simulink model "LIFT"  (R2019b)
settings: Solver=VariableStepAuto  StartTime=0.0  StopTime=inf  RelTol=1e-3
settings Model: Creator=u1830311  LastModifiedBy=u1830311

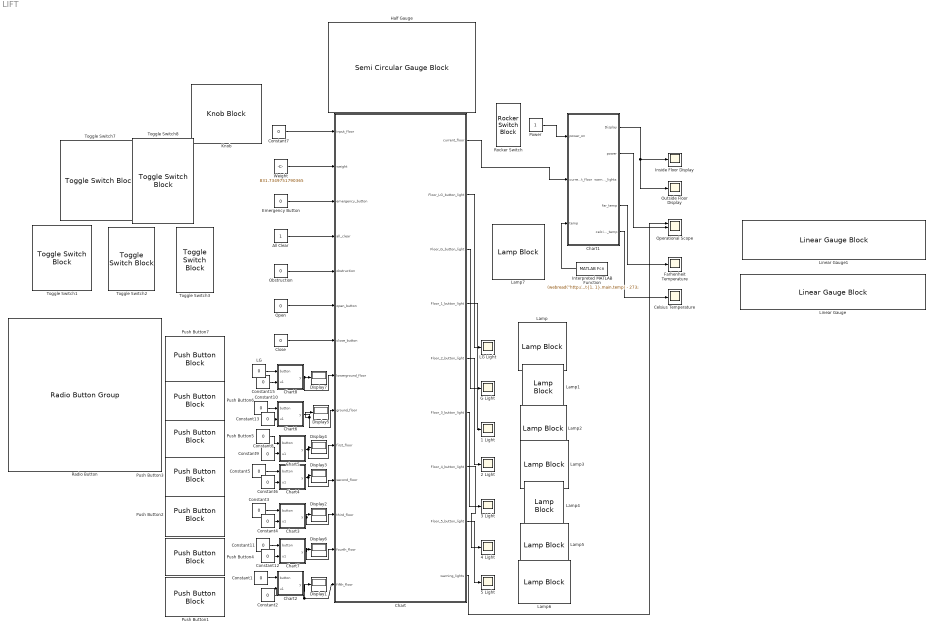
== system LIFT ==
  1 Light : Scope
  2 Light : Scope
  3 Light : Scope
  4 Light : Scope
  5 Light : Scope
  All Clear : Constant
  Celsius Temperature : Scope
  Chart : Stateflow chart  TreatAsAtomicUnit=on
  Chart1 : Stateflow chart  BlockKeywords=__PRM__SERIALIZED__DATA__:Stateflow Chart,Stateflow Diagram  TreatAsAtomicUnit=on
  Chart2 : Stateflow chart  BlockKeywords=__PRM__SERIALIZED__DATA__:Stateflow Chart,Stateflow Diagram  TreatAsAtomicUnit=on
  Chart3 : Stateflow chart  BlockKeywords=__PRM__SERIALIZED__DATA__:Stateflow Chart,Stateflow Diagram  TreatAsAtomicUnit=on
  Chart4 : Stateflow chart  BlockKeywords=__PRM__SERIALIZED__DATA__:Stateflow Chart,Stateflow Diagram  TreatAsAtomicUnit=on
  Chart5 : Stateflow chart  BlockKeywords=__PRM__SERIALIZED__DATA__:Stateflow Chart,Stateflow Diagram  TreatAsAtomicUnit=on
  Chart6 : Stateflow chart  BlockKeywords=__PRM__SERIALIZED__DATA__:Stateflow Chart,Stateflow Diagram  TreatAsAtomicUnit=on
  Chart7 : Stateflow chart  BlockKeywords=__PRM__SERIALIZED__DATA__:Stateflow Chart,Stateflow Diagram  TreatAsAtomicUnit=on
  Chart8 : Stateflow chart  BlockKeywords=__PRM__SERIALIZED__DATA__:Stateflow Chart,Stateflow Diagram  TreatAsAtomicUnit=on
  Close : Constant  Value=0
  Constant{1..13,15} (14 alike) : Constant  Value=0
  Display{1..7} (7 alike) : Display
  Emergency Button : Constant  Value=0
  Farhenheit Temperature : Scope
  G Light : Scope
  Half Gauge : SemiCircularGaugeBlock  ScaleMin=-1  ScaleMax=5  TickInterval=1
  "Inside Floor Display " : Scope
  Interpreted MATLAB Function : MATLABFcn  MATLABFcn="(webread(\"http://api.openweathermap.org/data/2.5/forecast?id=2652221&APPID=0d4add3479401fba2717516fc46e760f\").list{1, 1}.main.temp) - 273;"  OutputDimensions=1
  Knob : KnobBlock  ScaleMax=2000
  LG : Constant  Value=0
  LG Light : Scope
  Lamp{,1..7} (8 alike) : LampBlock
  Linear Gauge : LinearGaugeBlock  ScaleMin=-10  ScaleMax=50
  Linear Gauge1 : LinearGaugeBlock  ScaleMin=14  ScaleMax=122
  Obstruction : Constant  Value=0
  Open : Constant  Value=0
  "Operational Scope " : Scope  NumInputPorts=3
  "Outside Floor Display " : Scope
  Power : Constant
  Push Button1 : PushButtonBlock  ButtonText=5
  Push Button2 : PushButtonBlock  ButtonText=3
  Push Button3 : PushButtonBlock  ButtonText=2
  Push Button4 : PushButtonBlock  ButtonText=4
  Push Button5 : PushButtonBlock  ButtonText=1
  Push Button6 : PushButtonBlock  ButtonText=G
  Push Button7 : PushButtonBlock  ButtonText=LG
  Radio Button : RadioButtonGroup  SelectedLabel=Ground  ButtonGroupName=Start Floor
      settings: Values={{'Lower Ground', 'Ground', '1', '2', '3', '4', '5'}, [-1 0 1 2 3 4 5]}
  Rocker Switch : RockerSwitchBlock
      settings: Values={{'Off', 'On'}, [0 1]}
  Toggle Switch{1..3,7..8} (5 alike) : ToggleSwitchBlock
      settings: Values={{'Off', 'On'}, [0 1]}
  "Weight " : Constant  Value=831.7349751790365
  wires:
  Chart/1(current_floor) -> Chart1/2(current_floor)
  Constant7/1 -> Chart/1(input_floor)
  Power/1 -> Chart1/1(power_on)
  Chart1/2(power) -> "Operational Scope "/2
  Chart1/1(Display) -> "Outside Floor Display "/1, "Inside Floor Display "/1
  Chart1/4(far_temp) -> Farhenheit Temperature/1
  Chart1/5(celcius_temp) -> Celsius Temperature/1
  Chart/4(Floor_1_button_light) -> 1 Light/1
  Chart/5(Floor_2_button_light) -> 2 Light/1
  Chart/6(Floor_3_button_light) -> 3 Light/1
  Chart/7(Floor_4_button_light) -> 4 Light/1
  Chart/8(Floor_5_button_light) -> 5 Light/1
  All Clear/1 -> Chart/4(all_clear)
  "Weight "/1 -> Chart/2(weight)
  Emergency Button/1 -> Chart/3(emergency_button)
  Chart/9(warning_lights) -> "Operational Scope "/1
  Chart/3(Floor_G_button_light) -> G Light/1
  Chart/2(Floor_LG_button_light) -> LG Light/1
  Constant11/1 -> Chart7/1(button)
  Chart7/1(y) -> Display6/1, Chart/13(fourth_floor)
  Constant12/1 -> Chart7/2(u1)
  Constant2/1 -> Chart2/2(u1)
  Chart2/1(y) -> Display1/1, Chart/14(fifth_floor)
  Constant1/1 -> Chart2/1(button)
  Chart3/1(y) -> Display2/1, Chart/12(third_floor)
  Constant4/1 -> Chart3/2(u1)
  Constant3/1 -> Chart3/1(button)
  Chart4/1(y) -> Display3/1, Chart/11(second_floor)
  Constant6/1 -> Chart4/2(u1)
  Constant5/1 -> Chart4/1(button)
  Chart5/1(y) -> Chart/10(first_floor), Display4/1
  Constant8/1 -> Chart5/1(button)
  Chart6/1(y) -> Display5/1, Chart/9(ground_floor)
  Constant13/1 -> Chart6/2(u1)
  Constant10/1 -> Chart6/1(button)
  Chart8/1(y) -> Chart/8(lowerground_floor), Display7/1
  Constant15/1 -> Chart8/2(u1)
  LG/1 -> Chart8/1(button)
  Constant9/1 -> Chart5/2(u1)
  Obstruction/1 -> Chart/5(obstruction)
  Close/1 -> Chart/7(close_button)
  Open/1 -> Chart/6(open_button)
  Interpreted MATLAB Function/1 -> Chart1/3(temp)

== stateflow chart LIFT/Chart ==
  state Update_F2
    Floors(4) = 1;
  state Update_F4
    Floors(6) = 1;
  state Update_G
    Floors(2) = 1;
  state Update_F1
    Floors(3) = 1;
  state Update_F3
    Floors(5) = 1;
  state Update_F5
    Floors(7) = 1;
  state Update_LG
    Floors(1) = 1;
  state Moving
    entry:
    music=1;
    disp("music plays")
    during:
    if emergency_button == 1 || weight >= 1500
    emergency = 1;
    end
    state Up
      entry:
      if Floors(1)==1
      Floor_LG_button_light=1;
      end
      if Floors(2)==1
      Floor_G_button_light=1;
      end
      if Floors(3)==1
      Floor_1_button_light=1;
      end
      if Floors(4)==1
      Floor_2_button_light=1;
      end
      if Floors(5)==1
      Floor_3_button_light=1;
      end
      if Floors(6)==1
      Floor_4_button_light=1;
      end
      if Floors(7)==1
      Floor_5_button_light=1;
      end
      move=0;
      i=1;
      for(j=(current_floor+2):1:7)
      if (Floors(j)==1)
      up=1;
      break
      else
      up=0;
      end
      end
      during:
      for(j=(current_floor+2):1:7)
      if (Floors(j)==1)
      up=1;
      break
      else
      up=0;
      end
      end
      for (l=-1:1:4)
      while current_floor==l
      for(i=current_floor+2:1:7)
      if(Floors(i)==1)
      move=1;
      break
      end
      end
      break
      end
      end
    state Down
      entry:
      move=0;k=7;
      for(j=(current_floor+2):1:1)
      if (Floors(j)==1)
      up=0;
      break
      else
      up=1;
      end
      end
      during:
      for(m=5:-1:0)
      while current_floor==m
      for(k=current_floor+2:-1:1)
      if(Floors(k)==1)
      move=1;
      break
      end
      end
      break
      end
      end
    state Transport
      entry:
      if up==1
      current_floor=i-2;
      else
      current_floor=k-2;
      end
      if current_floor==-1
      Floor_LG_button_light=0;
      elseif current_floor==0
      Floor_G_button_light=0;
      elseif current_floor==1
      Floor_1_button_light=0;
      elseif current_floor==2
      Floor_2_button_light=0;
      elseif current_floor==3
      Floor_3_button_light=0;
      elseif current_floor==4
      Floor_4_button_light=0;
      elseif current_floor==5
      Floor_5_button_light=0;
      end
      exit:
      if up==1
      Floors(i)=0;
      else
      Floors(k)=0;
      end
      state Open_door
        entry:
        door_state=1;
        music = 0;
        sound = 1;
        switch current_floor
        case (-1)
        disp("Announcer: lower ground floor")
        disp("opening lower ground doors")
        case 0
        disp("Announcer: ground floor")
        disp("opening ground floor doors")
        case 1
        disp("Announcer: floor 1")
        disp("opening floor 1 doors")
        case 2
        disp("Announcer: floor 2")
        disp("opening floor 2 doors")
        case 3
        disp("Announcer: floor 3")
        disp("opening floor 3 doors")
        case 4
        disp("Announcer: floor 4")
        disp("opening floor 4 doors")
        case 5
        disp("Announcer: floor 5")
        disp("opening floor 5 doors")
        end
        sound = 0;
        pause(1)
        if door_state == 1
        disp("doors opening ")
        end
        during:
        tic
        while (toc<10)
        if obstruction == 1
        break
        end
        if close_button == 1
        break
        end
        if open_button == 1
        break
        end
        end
        exit:
      state Idle1
        entry:
        pause(3);
        door_state = 1;
        move=0;
      state Close_Door
        % Closes door
        during:
        pause(3);
        door_state = 0;
        sound = 1;
        if door_state == 0
        disp("Announcer: doors closing")
        switch current_floor
        case (-1)
        disp("system.out closing lower ground doors")
        case 0
        disp("system.out closing ground floor doors")
        case 1
        disp("system.out closing floor 1 doors")
        case 2
        disp("system.out closing floor 2 doors")
        case 3
        disp("system.out closing floor 3 doors")
        case 4
        disp("system.out closing floor 4 doors")
        case 5
        disp("system.out closing floor 5 doors")
        end
        end
        pause(2)
        music = 1;
        disp("music plays")
      (default) -> Idle1
      Idle1 -> Open_door : [move == 0]
      Open_door -> Open_door [order 1] : [open_button == 1 || obstruction == 1]
      Open_door -> Close_Door [order 2] : [(obstruction == 0 && open_button == 0) || close_button == 1]
    (default) -> Up
    Up -> Down [order 1] : [up==0]
    Down -> Up [order 1] : [up==1]
    Down -> Transport [order 2] : [move==1]
    Transport -> Down [order 2] : [move==0&&up==0&&door_state==0]
    Up -> Transport [order 2] : [move==1]
    Transport -> Up [order 1] : [move==0&&up==1&&door_state==0]
  state Input
    entry:
    Floors=[ lowerground_floor ground_floor first_floor second_floor third_floor fourth_floor fifth_floor ]'
    current_floor=input_floor;
    emergency = 0;
    Original=Floors
    during:
    Floors=[ lowerground_floor ground_floor first_floor second_floor third_floor fourth_floor fifth_floor ]'
  state Idle
    entry:
    music=0;
    door_state=1;
    exit:
    door_state=0;
    during:
    if [Floors(1)==0&&Floors(2)==0&&Floors(3)==0&&Floors(4)==0&&Floors(5)==0&&Floors(6)==0&&Floors(7)==0]
    Floors=[ lowerground_floor ground_floor first_floor second_floor third_floor fourth_floor fifth_floor ]'
    end
    exit:
    if Floors==Original
    Floors(1)=0;
    Floors(2)=0;
    Floors(3)=0;
    Floors(4)=0;
    Floors(5)=0;
    Floors(6)=0;
    Floors(7)=0;
    end
  state STOP
    entry:
    warning_lights = 1;
    during:
    if all_clear == 1 && weight < 1500 && emergency_button == 0
    emergency = 0;
    end
    exit:
    warning_lights = 0;
  (junction 293) -> (junction 298)
  Idle -> (junction 293) [order 8] : [hasChanged(fifth_floor)]
  (junction 298) -> Update_F5
  (junction 276) -> (junction 297)
  Idle -> (junction 276) [order 7] : [hasChanged(fourth_floor)]
  (junction 297) -> Update_F4
  (junction 275) -> (junction 296)
  Idle -> (junction 275) [order 6] : [hasChanged(third_floor)]
  (junction 296) -> Update_F3
  (junction 271) -> (junction 274)
  Idle -> (junction 271) [order 5] : [hasChanged(second_floor)]
  (junction 274) -> Update_F2
  (junction 270) -> (junction 273)
  Idle -> (junction 270) [order 4] : [hasChanged(first_floor)]
  (junction 273) -> Update_F1
  (junction 269) -> (junction 272)
  Idle -> (junction 269) [order 3] : [hasChanged(ground_floor)]
  (junction 272) -> Update_G
  (junction 277) -> (junction 278)
  Idle -> (junction 277) [order 2] : [hasChanged(lowerground_floor)]
  (junction 278) -> Update_LG
  Moving -> Update_F2 [order 6] : [hasChanged(second_floor)]
  Update_F2 -> Moving
  Moving -> Update_F4 [order 4] : [hasChanged(fourth_floor)]
  Update_F4 -> Moving
  Moving -> Update_G [order 9] : [hasChanged(ground_floor)]
  Update_G -> Moving
  Moving -> Update_F1 [order 2] : [hasChanged(first_floor)]
  Update_F1 -> Moving
  Moving -> Update_F3 [order 5] : [hasChanged(third_floor)]
  Update_F3 -> Moving
  Moving -> Update_F5 [order 3] : [hasChanged(fifth_floor)]
  Update_F5 -> Moving
  Moving -> Update_LG [order 8] : [hasChanged(lowerground_floor)]
  Update_LG -> Moving
  (default) -> Input
  Input -> Moving : [Floors(1)==1||Floors(2)==1||Floors(3)==1||Floors(4)==1||Floors(5)==1||Floors(6)==1||Floors(7)==1]
  Idle -> Moving [order 1] : [Floors(1)==1||Floors(2)==1||Floors(3)==1||Floors(4)==1||Floors(5)==1||Floors(6)==1||Floors(7)==1]
  Moving -> Idle [order 1] : [Floors(1)==0&&Floors(2)==0&&Floors(3)==0&&Floors(4)==0&&Floors(5)==0&&Floors(6)==0&&Floors(7)==0]
  Idle -> STOP [order 9] : [emergency_button == 1]
  Moving -> STOP [order 7] : [emergency ==1]
  STOP -> Idle : [emergency == 0]
  data: input_floor input; weight input; emergency_button input; all_clear input; obstruction input; open_button input; close_button input; lowerground_floor input; ground_floor input; current_floor output =-1; Floor_LG_button_light output =0; Floor_G_button_light output; first_floor input; second_floor input; third_floor input; i local; up local; move local; j local; k local; fourth_floor input; fifth_floor input; door_state local; Floors local; sound local; music local; Floor_1_button_light output; Floor_2_button_light output; Floor_3_button_light output; Floor_4_button_light output; Floor_5_button_light output; emergency local; warning_lights output; Original local; l local; m local

== stateflow chart LIFT/Chart2 ==
  state In1
    a = u1
  state In
  state Out
    entry:
    y = a + 1;
    exit:
    a = y
  (default) -> In1
  In1 -> In
  In -> Out : [hasChanged(button)]
  Out -> In
  data: button input; y output; u1 input; a local

== stateflow chart LIFT/Chart1 ==
  state On
    entry:
    power = 1
    during:
    celcius_temp = temp;
    far_temp = (celcius_temp .* (9/5) + 32);
    switch current_floor
    case -1
    Display = -1;
    case 0
    Display = 0;
    case 1
    Display = 1;
    case 2
    Display = 2;
    case 3
    Display = 3;
    case 4
    Display = 4;
    case 5
    Display = 5;
    otherwise
    Display = 00;
    emergency = 1;
    end % end switch
  state Off
    entry:
    power = 0;
    exit:
    emergency = 0;
  state Emergency
    entry:
    warning_lights = 1;
    exit:
    warning_lights = 0;
  (default) -> Off
  Off -> On : [power_on == 1]
  On -> Off [order 2] : [power_on == 0]
  Emergency -> On : [emergency == 0]
  On -> Emergency [order 1] : [emergency == 1]
  data: power_on input; Display output; power output; emergency local; current_floor input; warning_lights output; far_temp output; celcius_temp output; temp input

== stateflow chart LIFT/Chart3 ==
  state In1
    a = u1
  state In
  state Out
    entry:
    y = a + 1;
    exit:
    a = y
  (default) -> In1
  In1 -> In
  In -> Out : [hasChanged(button)]
  Out -> In
  data: button input; y output; u1 input; a local

== stateflow chart LIFT/Chart4 ==
  state In1
    a = u1
  state In
  state Out
    entry:
    y = a + 1;
    exit:
    a = y
  (default) -> In1
  In1 -> In
  In -> Out : [hasChanged(button)]
  Out -> In
  data: button input; y output; u1 input; a local

== stateflow chart LIFT/Chart5 ==
  state In1
    a = u1
  state In
  state Out
    entry:
    y = a + 1;
    exit:
    a = y
  (default) -> In1
  In1 -> In
  In -> Out : [hasChanged(button)]
  Out -> In
  data: button input; y output; u1 input; a local

== stateflow chart LIFT/Chart6 ==
  state In1
    a = u1
  state In
  state Out
    entry:
    y = a + 1;
    exit:
    a = y
  (default) -> In1
  In1 -> In
  In -> Out : [hasChanged(button)]
  Out -> In
  data: button input; y output; u1 input; a local

== stateflow chart LIFT/Chart7 ==
  state In1
    a = u1
  state In
  state Out
    entry:
    y = a + 1;
    exit:
    a = y
  (default) -> In1
  In1 -> In
  In -> Out : [hasChanged(button)]
  Out -> In
  data: button input; y output; u1 input; a local

== stateflow chart LIFT/Chart8 ==
  state In1
    a = u1
  state In
  state Out
    entry:
    y = a + 1;
    exit:
    a = y
  (default) -> In1
  In1 -> In
  In -> Out : [hasChanged(button)]
  Out -> In
  data: button input; y output; u1 input; a local
